simulink model "galvo_simulink"  (R2021a)
settings: Solver=VariableStepAuto  StartTime=0.0  StopTime=5  RelTol=1e-3
settings Model: Creator=TheCaT  LastModifiedBy=TheCaT

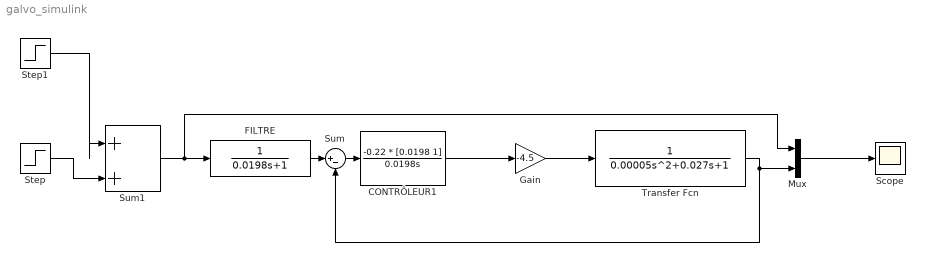
== system galvo_simulink ==
  CONTRÔLEUR1 : TransferFcn  Numerator=-0.22 * [0.0198 1]  Denominator=[0.0198 0]
  FILTRE : TransferFcn  Numerator=1  Denominator=[0.0198 1]
  Gain : Gain  Gain=-4.5
  Mux : Mux  Inputs=2
  Scope : Scope
  Step : Step  SampleTime=0
  Step1 : Step  Time=3  SampleTime=0
  Sum : Sum  Inputs=|+-
  Sum1 : Sum  Inputs=|++
  Transfer Fcn : TransferFcn  Denominator=[0.00005 0.027 1]
  wires:
  FILTRE/1 -> Sum/1
  Mux/1 -> Scope/1
  Transfer Fcn/1 -> Sum/2, Mux/2
  Sum/1 -> CONTRÔLEUR1/1
  Sum1/1 -> Mux/1, FILTRE/1
  Step/1 -> Sum1/2
  Step1/1 -> Sum1/1
  Gain/1 -> Transfer Fcn/1
  CONTRÔLEUR1/1 -> Gain/1
